simulink model "p1_standalone"  (R2014a)
settings: Solver=ode1  SolverMode=SingleTasking  StartTime=0  StopTime=36000  FixedStep=Ts  RelTol=1e-3
PreLoadFcn:
  | InitModel
  | make
InitFcn:
  | InitModel
  | make
values from neighbouring files (symbols this model uses):
  num = num+MTnum(m)    [Build_MtMuMy.m]
  Ts = 0.002    [DSC_Control_Analysis.m]    (also in DSC_Control_Analysis_Exp.m; DSC_Speed_Control_Analysis.m; EC_params_nissan.m; Ext_MPCPara.m = SSD.Ts)
undefined symbols (not defined in the file or in its folder): den, DiscIntNeverNeededParam, gpsins, gr, hal_filter_den, hal_filter_num, Igain_l, Igain_r, Imax_l, Imax_r, Ioff_l, Ioff_r, KB, Kd, KF, Ki, KJ, Kp, param, sglu
libraries: simulink x5, slrtlib x3, xpcdiamondlib x2, UserBlocks x1
(part 2 of 3)

== system p1_standalone/Hardware I//O/Input/GPS Velocity and Position ==
  Demux : Demux  Outputs=19
  GPS Velocity : S-Function  FunctionName=rs232_OEM4_MultiMode  Parameters=Ts, ModeSelect  EnableBusSupport=off
  Mux : Mux  Inputs=19
  Raw GPS : Outport
  wires:
  Mux/1 -> Raw GPS/1
  Demux/6 -> Mux/6  "Velocity Status Vel"
  Demux/7 -> Mux/7  "UTC DGPS"
  Demux/5 -> Mux/5  "Vert Speed"
  Demux/4 -> Mux/4  "Horiz Speed Direction"
  Demux/3 -> Mux/3  "Horiz Speed"
  Demux/2 -> Mux/2  "Latency Vel"
  Demux/1 -> Mux/1  "UTC Vel"
  Demux/19 -> Mux/19  "Latency"
  Demux/18 -> Mux/18  "Num Satellites"
  Demux/17 -> Mux/17  "Velocity z"
  Demux/16 -> Mux/16  "Velocity y"
  Demux/15 -> Mux/15  "Velocity x"
  Demux/14 -> Mux/14  "Velocity Solution Type"
  Demux/13 -> Mux/13  "Velocity Status"
  Demux/12 -> Mux/12  "Position z"
  Demux/11 -> Mux/11  "Postion y"
  Demux/10 -> Mux/10  "Position x"
  Demux/9 -> Mux/9  "Position Solution Type"
  Demux/8 -> Mux/8  "Position Status"
  GPS Velocity/1 -> Demux/1

== system p1_standalone/Hardware I//O/Input/Gearbox angle scaling ==
  raw gb angles : Inport
  Pot readings with wheels centered : Constant  Value=[ -1.73; -3.56 ]
  Sum : Sum  Inputs=|++  SaturateOnIntegerOverflow=on
  Volts/Rad : Gain  Gain=[1/ -1.31; 1/-1.34]  SaturateOnIntegerOverflow=on  OutDataTypeStr=Inherit: Same as input  ParamDataTypeStr=Inherit: Same as input
  gb angles : Outport
  wires:
  Volts/Rad/1 -> gb angles/1
  Pot readings with wheels centered/1 -> Sum/2
  raw gb angles/1 -> Sum/1
  Sum/1 -> Volts/Rad/1

== system p1_standalone/Hardware I//O/Input/Handwheel Scaling & Initialization ==
  Relative : Inport
  Absolute : Inport  Port=2
  Encoder Initialization : Subsystem
  Handwheel Gear Ratio : Gain  Gain=(60/18)*50  SaturateOnIntegerOverflow=on  OutDataTypeStr=Inherit: Same as input  ParamDataTypeStr=Inherit: Same as input
  Handwheel Sensor Fault Detection : Subsystem
  Harmonic Drive Gear Ratio : Gain  Gain=1/50  SaturateOnIntegerOverflow=on  OutDataTypeStr=Inherit: Same as input  ParamDataTypeStr=Inherit: Same as input
  Harmonic Drive Gear Ratio1 : Gain  Gain=1/50  SaturateOnIntegerOverflow=on  OutDataTypeStr=Inherit: Same as input  ParamDataTypeStr=Inherit: Same as input
  Sum : Sum  Inputs=|++
  encoder scaling : Gain  Gain=2*pi/(4*500)  SaturateOnIntegerOverflow=on  OutDataTypeStr=Inherit: Same as input  ParamDataTypeStr=Inherit: Same as input
  handwheel offset : Constant  Value=-1.29*pi/180*10
  Primary : Outport
  Secondary : Outport  Port=2
  Fault : Outport  Port=3
  wires:
  encoder scaling/1 -> Encoder Initialization/1(Relative Encoder)  "Primary"
  Handwheel Gear Ratio/1 -> Encoder Initialization/2(Absolute Encoder), Harmonic Drive Gear Ratio1/1
  Handwheel Sensor Fault Detection/3(Fault) -> Fault/1  "Encoder Fault Status"
  Encoder Initialization/1(Calibrated) -> Harmonic Drive Gear Ratio/1
  Handwheel Sensor Fault Detection/2(Secondary) -> Secondary/1  "Secondary"
  Harmonic Drive Gear Ratio/1 -> Handwheel Sensor Fault Detection/1(Relative)
  Relative/1 -> encoder scaling/1
  Absolute/1 -> Handwheel Gear Ratio/1
  Harmonic Drive Gear Ratio1/1 -> Handwheel Sensor Fault Detection/2(Absolute)
  handwheel offset/1 -> Sum/1
  Sum/1 -> Primary/1
  Handwheel Sensor Fault Detection/1(Primary) -> Sum/2  "Primary"

== system p1_standalone/Hardware I//O/Input/INS scaling ==
  raw INS : Inport
  Bus Creator : BusCreator  Inputs=6
  Demux : Demux  Outputs=9
  Gain : Gain  Gain=9.81  SaturateOnIntegerOverflow=on  OutDataTypeStr=Inherit: Same as input  ParamDataTypeStr=Inherit: Same as input
  Gain1 : Gain  Gain=1/.018  SaturateOnIntegerOverflow=on  OutDataTypeStr=Inherit: Same as input  ParamDataTypeStr=Inherit: Same as input
  Gain2 : Gain  Gain=1/.018  SaturateOnIntegerOverflow=on  OutDataTypeStr=Inherit: Same as input  ParamDataTypeStr=Inherit: Same as input
  Gain3 : Gain  Gain=9.81  SaturateOnIntegerOverflow=on  OutDataTypeStr=Inherit: Same as input  ParamDataTypeStr=Inherit: Same as input
  Gain4 : Gain  Gain=9.81  SaturateOnIntegerOverflow=on  OutDataTypeStr=Inherit: Same as input  ParamDataTypeStr=Inherit: Same as input
  Gain5 : Gain  Gain=1/.018  SaturateOnIntegerOverflow=on  OutDataTypeStr=Inherit: Same as input  ParamDataTypeStr=Inherit: Same as input
  Sum{,1..5} (6 alike) : Sum  Inputs=+-  SaturateOnIntegerOverflow=on  InputSameDT=on  OutDataTypeStr=Inherit: Same as first input
  deg to rad : Gain  Gain=pi/180  SaturateOnIntegerOverflow=on  OutDataTypeStr=Inherit: Same as input  ParamDataTypeStr=Inherit: Same as input
  INS : Outport
  wires:
  Demux/6 -> Sum2/2, Sum/2
  Demux/4 -> Sum2/1
  Demux/2 -> Sum3/1
  Demux/3 -> Sum3/2, Sum1/2
  Demux/1 -> Sum1/1
  Gain3/1 -> Bus Creator/2  "ax"
  Gain2/1 -> Bus Creator/3  "roll"
  Gain1/1 -> deg to rad/1  "yaw rate"
  Gain/1 -> Bus Creator/4  "ay"
  Sum3/1 -> Gain3/1
  Sum2/1 -> Gain2/1
  Sum1/1 -> Gain1/1
  Sum/1 -> Gain/1
  raw INS/1 -> Demux/1
  Gain5/1 -> Bus Creator/5  "pitch"
  Gain4/1 -> Bus Creator/6  "az"
  Sum5/1 -> Gain5/1
  Sum4/1 -> Gain4/1
  Demux/7 -> Sum5/1
  Demux/8 -> Sum4/1
  Demux/5 -> Sum/1
  Demux/9 -> Sum5/2, Sum4/2
  deg to rad/1 -> Bus Creator/1  "yaw"
  Bus Creator/1 -> INS/1

== system p1_standalone/Hardware I//O/Input/OEM4 wgsxyz2enu and status conversion ==
  raw GPS : Inport
  Bus Creator : BusCreator  Inputs=6
  Bus Creator1 : BusCreator  Inputs=6
  Bus Creator2 : BusCreator  Inputs=2
  Bus Creator3 : BusCreator  Inputs=6
  Bus Creator4 : BusCreator  Inputs=3
  Demux : Demux  Outputs=19
  Gain to make CW : Gain  Gain=-1
  Mode Select : Constant
  Switch : Switch  Threshold=0.5
  position preprocessing : Subsystem
  velocity preprocessing : Subsystem
  OEM4 Velocity : Outport
  OEM4 position : Outport  Port=2
  OEM4 other : Outport  Port=3
  OEM4 rawXYZ : Outport  Port=4
  wires:
  Switch/1 -> OEM4 Velocity/1
  Mode Select/1 -> Switch/2
  Bus Creator3/1 -> Switch/1
  Demux/6 -> Bus Creator3/6  "Velocity Solution Status"
  Demux/5 -> Bus Creator3/5  "Vertical Speed"
  Demux/4 -> Bus Creator3/4  "Horizontal Velocity Direction"
  Demux/3 -> Bus Creator3/3  "Horizontal Speed"
  Demux/2 -> Bus Creator3/2  "Latency"
  Demux/1 -> Bus Creator3/1  "UTC"
  Demux/19 -> Bus Creator1/2  "Latency"
  Gain to make CW/1 -> Bus Creator1/4  "Horizontal Velocity Direction"
  Demux/14 -> Bus Creator2/1  "Velocity Solution Type"
  Demux/18 -> Bus Creator2/2  "Number Of Satellites"
  Bus Creator2/1 -> OEM4 other/1
  Bus Creator/1 -> OEM4 position/1
  Demux/7 -> Bus Creator1/1, Bus Creator/1  "UTC"
  position preprocessing/3(Pos Up (z)) -> Bus Creator/6  "Pos Up (z)"
  position preprocessing/2(Pos N (y)) -> Bus Creator/5  "Pos N (y)"
  position preprocessing/1(Pos E (x)) -> Bus Creator/4  "Pos E (x)"
  Demux/8 -> Bus Creator/2  "Position Solution Status"
  Demux/9 -> Bus Creator/3  "Position Solution Type"
  Demux/10 -> position preprocessing/1(Pos x), Bus Creator4/1  "GPS_rawX"
  Demux/11 -> position preprocessing/2(Pos y), Bus Creator4/2  "GPS_rawY"
  Demux/12 -> position preprocessing/3(Pos z), Bus Creator4/3  "GPS_rawZ"
  velocity preprocessing/1(horizontal speed) -> Bus Creator1/3  "Horizontal Speed"
  velocity preprocessing/2(velocity direction) -> Gain to make CW/1  "Horizontal Velocity Direction"
  velocity preprocessing/3(vertical speed) -> Bus Creator1/5  "Vertical Speed"
  velocity preprocessing/4(velocity status) -> Bus Creator1/6  "Velocity Solution Status"
  Demux/13 -> velocity preprocessing/1(Vel status)
  Demux/15 -> velocity preprocessing/2(Vel x)  "Velocity Solution Type"
  Demux/16 -> velocity preprocessing/3(Vel y)
  Demux/17 -> velocity preprocessing/4(Vel z)
  Bus Creator1/1 -> Switch/3
  raw GPS/1 -> Demux/1
  Bus Creator4/1 -> OEM4 rawXYZ/1

== system p1_standalone/Hardware I//O/Input/Rear Wheel Speed Processing ==
  ticks : Inport
  Demux : Demux  Outputs=2
  Mux : Mux  Inputs=2
  Speed Calc : Subsystem  mask{range=65536}
      mask prompts: range "Wrap range"
      mask Display: disp(range);
  Speed Calc1 : Subsystem  mask{range=65536}
      mask prompts: range "Wrap range"
      mask Display: disp(range);
  de-quadrature : Gain  Gain=1/2
  ticks/sample : Outport
  wires:
  ticks/1 -> Demux/1
  Demux/1 -> Speed Calc/1(Distance)
  Speed Calc/1(Speed) -> Mux/1
  Demux/2 -> Speed Calc1/1(Distance)
  Speed Calc1/1(Speed) -> Mux/2
  Mux/1 -> de-quadrature/1
  de-quadrature/1 -> ticks/sample/1

== system p1_standalone/Hardware I//O/Input/Steering Motor Encoder Initialization ==
  Raw : Inport
  Potentiometer : Inport  Port=2
  Alignment : Inport  Port=3
  Demux : Demux  Outputs=2
  Demux1 : Demux  Outputs=2
  Left : Subsystem
  Mux : Mux  Inputs=2
  Right : Subsystem
  Sum1 : Sum  Inputs=++|
  Sum2 : Sum  Inputs=|++
  gearbox ratio : Gain  Gain=gr  SaturateOnIntegerOverflow=on  OutDataTypeStr=Inherit: Same as input  ParamDataTypeStr=Inherit: Same as input
  gearbox ratio1 : Gain  Gain=gr  SaturateOnIntegerOverflow=on  OutDataTypeStr=Inherit: Same as input  ParamDataTypeStr=Inherit: Same as input
  Angles : Outport
  Gearbox Angles : Outport  Port=2
  wires:
  Sum1/1 -> Gearbox Angles/1
  gearbox ratio1/1 -> Sum2/2
  Alignment/1 -> Sum1/1, gearbox ratio1/1
  Sum2/1 -> Angles/1
  Mux/1 -> Sum2/1
  Right/1(Calibrated) -> Mux/2
  gearbox ratio/1 -> Demux1/1
  Raw/1 -> Demux/1
  Potentiometer/1 -> Sum1/2, gearbox ratio/1
  Left/1(Calibrated) -> Mux/1
  Demux/1 -> Left/1(Encoder)
  Demux/2 -> Right/1(Encoder)
  Demux1/1 -> Left/2(Potentiometer)
  Demux1/2 -> Right/2(Potentiometer)

== system p1_standalone/Hardware I//O/Input/Subsystem1 ==
  In1 : Inport
  Constant : Constant
  Sum : Sum  Inputs=+-|
  Out1 : Outport
  wires:
  Sum/1 -> Out1/1
  In1/1 -> Sum/2
  Constant/1 -> Sum/1

== system p1_standalone/Hardware I//O/Input/Subsystem2 ==
  In1 : Inport
  Constant : Constant
  Sum : Sum  Inputs=+-|
  Out1 : Outport
  wires:
  Constant/1 -> Sum/1
  In1/1 -> Sum/2
  Sum/1 -> Out1/1

== system p1_standalone/Hardware I//O/Input/VSBC Analog Demux ==
  In : Inport
  Constant : Constant  Value=2.67
  Demux : Demux  Outputs=8
  Mux1 : Mux  Inputs=2
  Mux2 : Mux  Inputs=2
  Sum : Sum  Inputs=|+-
  T3 : Terminator
  Voltage to Rad : Gain  Gain=-(38.6)*(pi/180)
  PPS : Outport
  Motor Currents : Outport  Port=2
  HW Motor Current : Outport  Port=3
  HW Absolute Pot : Outport  Port=4
  Rear Load Cells : Outport  Port=5
  wires:
  Mux1/1 -> Motor Currents/1
  In/1 -> Demux/1
  Demux/7 -> Mux1/2
  Demux/6 -> Mux1/1
  Demux/3 -> HW Motor Current/1
  Demux/1 -> PPS/1
  Demux/8 -> T3/1
  Voltage to Rad/1 -> HW Absolute Pot/1
  Demux/4 -> Sum/1
  Sum/1 -> Voltage to Rad/1
  Constant/1 -> Sum/2
  Demux/2 -> Mux2/1
  Demux/5 -> Mux2/2
  Mux2/1 -> Rear Load Cells/1

== system p1_standalone/Hardware I//O/Input/current scaling ==
  volts : Inport
  Constant : Constant  Value=-5.39
  Sum : Sum  Inputs=|++  SaturateOnIntegerOverflow=on
  current scaling : Gain  Gain=30/7.5*3.3  SaturateOnIntegerOverflow=on  OutDataTypeStr=Inherit: Same as input  ParamDataTypeStr=Inherit: Same as input
  amps : Outport
  wires:
  volts/1 -> current scaling/1
  current scaling/1 -> Sum/1
  Sum/1 -> amps/1
  Constant/1 -> Sum/2

== system p1_standalone/Hardware I//O/Output/ConvertForce2Volt ==
  ForceDesired : Inport
  VoltDesired : Outport
  wires:
  ForceDesired/1 -> VoltDesired/1

== system p1_standalone/Sensor Data and Estimation/Nonlinear Observer/Normal Loads ==
  Vehicle States : Inport
  Bus Creator : BusCreator  Inputs=2
  Bus Selector1 : BusSelector  OutputSignals=Roll Angle,ayCG
  CG height : Constant  Value=0.49
  Fnf_nom : Constant  Value=param.m*9.81*param.b/(2*(param.a+param.b))
  Fnr_nom : Constant  Value=param.m*9.81*param.b/(2*(param.a+param.b))
  Front Mass : Constant  Value=param.m*param.b/(param.b+param.a)
  Left Normal Load : Sum  Inputs=+-
  Right Normal Load : Sum
  Roll Stiffness : Constant  Value=param.k_roll*0
  Saturation : Saturate  UpperLimit=deg2rad(8)  LowerLimit=-deg2rad(8)
  Track Width : Constant  Value=param.tw
  Track Width1 : Constant  Value=param.tw
  dFz : Sum
  dFz Ay Contribution : Product  Inputs=***/
  dFz Roll Contribution : Product  Inputs=**/
  Normal Loads : Outport
  wires:
  Bus Creator/1 -> Normal Loads/1
  Left Normal Load/1 -> Bus Creator/1  "Left"
  Right Normal Load/1 -> Bus Creator/2  "Right"
  Vehicle States/1 -> Bus Selector1/1
  Roll Stiffness/1 -> dFz Roll Contribution/1
  Bus Selector1/1 -> Saturation/1  "<Roll Angle>"
  Track Width1/1 -> dFz Roll Contribution/3
  Bus Selector1/2 -> dFz Ay Contribution/1  "<ayCG>"
  Front Mass/1 -> dFz Ay Contribution/2
  Fnf_nom/1 -> Left Normal Load/1
  dFz Roll Contribution/1 -> dFz/1
  dFz Ay Contribution/1 -> dFz/2
  dFz/1 -> Left Normal Load/2, Right Normal Load/1
  Fnr_nom/1 -> Right Normal Load/2
  Saturation/1 -> dFz Roll Contribution/2
  CG height/1 -> dFz Ay Contribution/3
  Track Width/1 -> dFz Ay Contribution/4

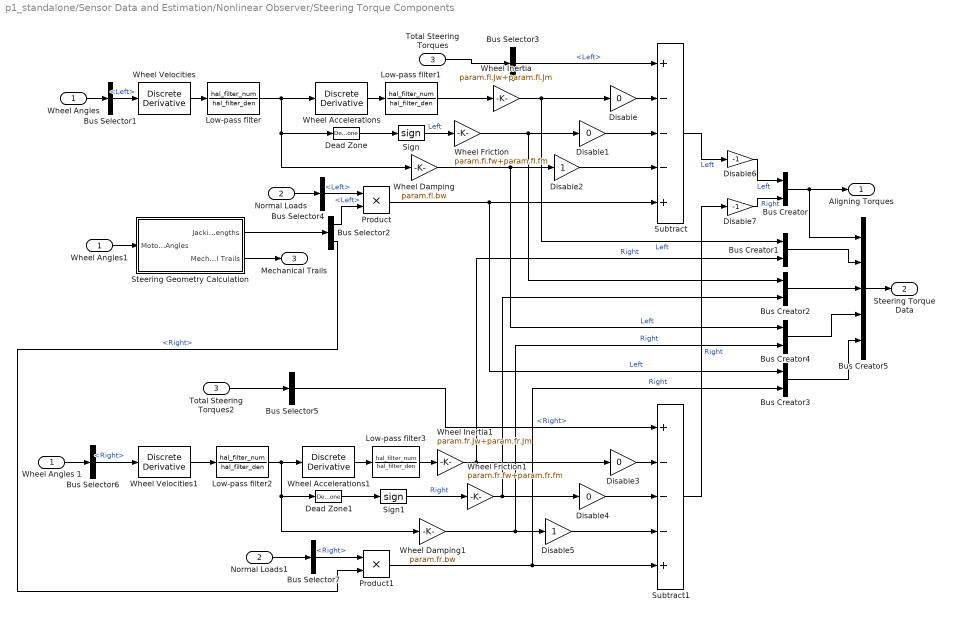
== system p1_standalone/Sensor Data and Estimation/Nonlinear Observer/Steering Torque Components ==
  Wheel Angles : Inport
  Normal Loads : Inport  Port=2
  Total Steering Torques : Inport  Port=3
  Bus Creator{,1..4} (5 alike) : BusCreator  Inputs=2
  Bus Creator5 : BusCreator  Inputs=5
  Bus Selector1 : BusSelector  OutputSignals=Left
  Bus Selector2 : BusSelector  OutputSignals=Left,Right
  Bus Selector3 : BusSelector  OutputSignals=Left
  Bus Selector4 : BusSelector  OutputSignals=Left
  Bus Selector5 : BusSelector  OutputSignals=Right
  Bus Selector6 : BusSelector  OutputSignals=Right
  Bus Selector7 : BusSelector  OutputSignals=Right
  Dead Zone : DeadZone  LowerValue=-0.03  UpperValue=0.03  SaturateOnIntegerOverflow=on
  Dead Zone1 : DeadZone  LowerValue=-0.03  UpperValue=0.03  SaturateOnIntegerOverflow=on
  Disable{,1,3..4} (4 alike) : Gain  Gain=0
  Disable2 : Gain
  Disable5 : Gain
  Disable6 : Gain  Gain=-1
  Disable7 : Gain  Gain=-1
  Low-pass filter{,1..3} (4 alike) : DiscreteTransferFcn  Numerator=hal_filter_num  Denominator=hal_filter_den  SampleTime=Ts
  Normal Loads1 : InportShadow  Port=2
  Product : Product  RndMeth=Zero
  Product1 : Product  RndMeth=Zero
  Sign : Signum
  Sign1 : Signum
  Steering Geometry Calculation : Subsystem
      mask init:
      | p1_params
      | nissan_steer_lookup_data
  Subtract : Sum  Inputs=+---+
  Subtract1 : Sum  Inputs=+---+
  Total Steering Torques2 : InportShadow  Port=3
  Wheel Accelerations : simulink/Discrete/Discrete Derivative  gainval=1.0  ICPrevScaledInput=0.0  InputProcessing=Inherited  OutMin=[]  OutMax=[]  OutDataType=sfix(16)  OutScaling=2^-10  DoSatur=off
  Wheel Accelerations1 : simulink/Discrete/Discrete Derivative  gainval=1.0  ICPrevScaledInput=0.0  InputProcessing=Inherited  OutMin=[]  OutMax=[]  OutDataType=sfix(16)  OutScaling=2^-10  DoSatur=off
  Wheel Angles 1 : InportShadow
  Wheel Angles1 : InportShadow
  Wheel Damping : Gain  Gain=param.fl.bw
  Wheel Damping1 : Gain  Gain=param.fr.bw
  Wheel Friction : Gain  Gain=param.fl.fw+param.fl.fm
  Wheel Friction1 : Gain  Gain=param.fr.fw+param.fr.fm
  Wheel Inertia : Gain  Gain=param.fl.Jw+param.fl.Jm
  Wheel Inertia1 : Gain  Gain=param.fr.Jw+param.fr.Jm
  Wheel Velocities : simulink/Discrete/Discrete Derivative  gainval=1.0  ICPrevScaledInput=0.0  InputProcessing=Inherited  OutMin=[]  OutMax=[]  OutDataType=sfix(16)  OutScaling=2^-10  DoSatur=off
  Wheel Velocities1 : simulink/Discrete/Discrete Derivative  gainval=1.0  ICPrevScaledInput=0.0  InputProcessing=Inherited  OutMin=[]  OutMax=[]  OutDataType=sfix(16)  OutScaling=2^-10  DoSatur=off
  Aligning Torques : Outport
  Steering Torque Data : Outport  Port=2
  Mechanical Trails : Outport  Port=3
  wires:
  Bus Selector3/1 -> Subtract/1  "<Left>"
  Wheel Velocities/1 -> Low-pass filter/1
  Steering Geometry Calculation/2(Mechanical Trails) -> Mechanical Trails/1
  Sign/1 -> Wheel Friction/1  "Left"
  Normal Loads/1 -> Bus Selector4/1
  Product/1 -> Bus Creator3/1, Subtract/5  "Left"
  Wheel Accelerations/1 -> Low-pass filter1/1
  Wheel Inertia/1 -> Bus Creator1/1, Disable/1  "Left"
  Wheel Angles/1 -> Bus Selector1/1
  Bus Selector5/1 -> Subtract1/1  "<Right>"
  Wheel Velocities1/1 -> Low-pass filter2/1
  Sign1/1 -> Wheel Friction1/1  "Right"
  Product1/1 -> Bus Creator3/2, Subtract1/5  "Right"
  Wheel Accelerations1/1 -> Low-pass filter3/1
  Wheel Inertia1/1 -> Bus Creator1/2, Disable3/1  "Right"
  Bus Selector1/1 -> Wheel Velocities/1  "<Left>"
  Bus Selector4/1 -> Product/1  "<Left>"
  Steering Geometry Calculation/1(Jacking Arm Lengths) -> Bus Selector2/1
  Bus Selector2/1 -> Product/2  "<Left>"
  Wheel Angles 1/1 -> Bus Selector6/1
  Bus Selector6/1 -> Wheel Velocities1/1  "<Right>"
  Bus Selector2/2 -> Product1/2  "<Right>"
  Normal Loads1/1 -> Bus Selector7/1
  Bus Selector7/1 -> Product1/1  "<Right>"
  Bus Creator/1 -> Aligning Torques/1, Bus Creator5/1
  Subtract/1 -> Disable6/1  "Left"
  Subtract1/1 -> Disable7/1  "Right"
  Wheel Damping/1 -> Bus Creator4/1, Disable2/1  "Left"
  Wheel Damping1/1 -> Bus Creator4/2, Disable5/1  "Right"
  Wheel Friction/1 -> Bus Creator2/1, Disable1/1
  Wheel Friction1/1 -> Bus Creator2/2, Disable4/1
  Bus Creator5/1 -> Steering Torque Data/1
  Bus Creator1/1 -> Bus Creator5/2
  Bus Creator2/1 -> Bus Creator5/3
  Bus Creator4/1 -> Bus Creator5/4
  Bus Creator3/1 -> Bus Creator5/5
  Disable/1 -> Subtract/2
  Disable1/1 -> Subtract/3
  Disable2/1 -> Subtract/4
  Disable3/1 -> Subtract1/2
  Disable4/1 -> Subtract1/3
  Disable5/1 -> Subtract1/4
  Total Steering Torques2/1 -> Bus Selector5/1
  Total Steering Torques/1 -> Bus Selector3/1
  Disable6/1 -> Bus Creator/1  "Left"
  Disable7/1 -> Bus Creator/2  "Right"
  Low-pass filter/1 -> Wheel Damping/1, Dead Zone/1, Wheel Accelerations/1
  Low-pass filter1/1 -> Wheel Inertia/1
  Low-pass filter2/1 -> Wheel Accelerations1/1, Wheel Damping1/1, Dead Zone1/1
  Low-pass filter3/1 -> Wheel Inertia1/1
  Dead Zone/1 -> Sign/1
  Dead Zone1/1 -> Sign1/1
  Wheel Angles1/1 -> Steering Geometry Calculation/1(Motor Angles)

== system p1_standalone/Sensor Data and Estimation/Steering Kinematics/Steer Torque Calculation ==
  Motor Angles : Inport
  Load Cells : Inport  Port=2
  Bus Creator : BusCreator  Inputs=2
  Demux : Demux  Outputs=2
  Demux1 : Demux  Outputs=2
  Left Arm Length Look-up : Lookup_n-D  NumberOfTableDimensions=1  BreakpointsForDimension1=sglu.fl.ma  Table=sglu.fl.lc  InternalRulePriority=Speed  SaturateOnIntegerOverflow=on  InputSameDT=on
  Left Steering Ratio : Gain  Gain=1/param.fl.gr  SaturateOnIntegerOverflow=on  OutDataTypeStr=Inherit: Same as input  ParamDataTypeStr=Inherit: Same as input
  Product : Product  RndMeth=Zero
  Product1 : Product  RndMeth=Zero
  Right Arm Length Look-up : Lookup_n-D  NumberOfTableDimensions=1  BreakpointsForDimension1=sglu.fr.ma  Table=sglu.fr.lc  InternalRulePriority=Speed  SaturateOnIntegerOverflow=on  InputSameDT=on
  Right Steering Ratio : Gain  Gain=1/param.fr.gr  SaturateOnIntegerOverflow=on  OutDataTypeStr=Inherit: Same as input  ParamDataTypeStr=Inherit: Same as input
  Steer Torques : Outport
  wires:
  Motor Angles/1 -> Demux/1
  Bus Creator/1 -> Steer Torques/1
  Demux/1 -> Left Steering Ratio/1
  Demux/2 -> Right Steering Ratio/1
  Left Steering Ratio/1 -> Left Arm Length Look-up/1
  Right Steering Ratio/1 -> Right Arm Length Look-up/1
  Load Cells/1 -> Demux1/1
  Demux1/2 -> Product1/2
  Demux1/1 -> Product/2
  Left Arm Length Look-up/1 -> Product/1
  Right Arm Length Look-up/1 -> Product1/1
  Product1/1 -> Bus Creator/2  "Right"
  Product/1 -> Bus Creator/1  "Left"

== system p1_standalone/Sensor Data and Estimation/Steering Kinematics/Steering Angle Calculation ==
  Motor Angles : Inport
  Bus Creator : BusCreator  Inputs=2
  Demux : Demux  Outputs=2
  Left Steer Angle Look-up : Lookup_n-D  NumberOfTableDimensions=1  BreakpointsForDimension1=sglu.fl.ma  Table=sglu.fl.sa  InternalRulePriority=Speed  SaturateOnIntegerOverflow=on  InputSameDT=on
  Left Steering Ratio : Gain  Gain=1/param.fl.gr  SaturateOnIntegerOverflow=on  OutDataTypeStr=Inherit: Same as input  ParamDataTypeStr=Inherit: Same as input
  Right Steer Angle Look-up : Lookup_n-D  NumberOfTableDimensions=1  BreakpointsForDimension1=sglu.fr.ma  Table=sglu.fr.sa  InternalRulePriority=Speed  SaturateOnIntegerOverflow=on  InputSameDT=on
  Right Steering Ratio : Gain  Gain=1/param.fr.gr  SaturateOnIntegerOverflow=on  OutDataTypeStr=Inherit: Same as input  ParamDataTypeStr=Inherit: Same as input
  Steer Angles : Outport
  wires:
  Motor Angles/1 -> Demux/1
  Bus Creator/1 -> Steer Angles/1
  Demux/1 -> Left Steering Ratio/1
  Demux/2 -> Right Steering Ratio/1
  Left Steering Ratio/1 -> Left Steer Angle Look-up/1
  Right Steering Ratio/1 -> Right Steer Angle Look-up/1
  Left Steer Angle Look-up/1 -> Bus Creator/1  "Left"
  Right Steer Angle Look-up/1 -> Bus Creator/2  "Right"

== system p1_standalone/Sensor Data and Estimation/Vehicle State Estimator/Select: Yaw Rate ==
  In1 : Inport
  Gain : Gain  Gain=K  Multiplication=Matrix(K*u)  SaturateOnIntegerOverflow=on  OutDataTypeStr=Inherit: Same as input  ParamDataTypeStr=Inherit: Same as input
  Out1 : Outport
  wires:
  Gain/1 -> Out1/1
  In1/1 -> Gain/1

== system p1_standalone/Sensor Data and Estimation/Vehicle State Estimator/state estimation ==
  gps : Inport
  ins : Inport  Port=2
  Bus Creator : BusCreator  Inputs=21
  DegtoRad{1..7} (7 alike) : Gain  Gain=pi/180
  Roll Gyro Sf : Constant
  Super Filter : Subsystem
  Filter Output : Outport
  wires:
  Super Filter/8(Vx) -> Bus Creator/9  "Vx"
  Super Filter/9(ax bias) -> Bus Creator/10  "ax bias"
  Super Filter/12(VyCG) -> Bus Creator/12  "VyCG"
  Super Filter/13(axCG) -> Bus Creator/11  "axCG"
  Bus Creator/1 -> Filter Output/1
  DegtoRad2/1 -> Bus Creator/1  "Yaw Angle"
  Super Filter/1(Yaw Angle) -> DegtoRad2/1  "Yaw Angle"
  Super Filter/4(Corr Yaw Rate) -> DegtoRad1/1  "Yaw Rate"
  DegtoRad1/1 -> Bus Creator/4  "Yaw Rate"
  Super Filter/5(Roll Angle) -> DegtoRad3/1  "Roll Angle"
  DegtoRad3/1 -> Bus Creator/5  "Roll Angle"
  Super Filter/7(Corr Roll Rate) -> DegtoRad4/1  "Roll Rate"
  DegtoRad4/1 -> Bus Creator/8  "Roll Rate"
  DegtoRad5/1 -> Bus Creator/3  "Yaw Gyro Bias"
  Super Filter/3(Yaw Gyro Bias) -> DegtoRad5/1  "Yaw Gyro Bias"
  Super Filter/6(Roll Gyro Bias) -> DegtoRad6/1  "Roll Gyro Bias"
  DegtoRad6/1 -> Bus Creator/7  "Roll Gyro Bias"
  DegtoRad7/1 -> Bus Creator/15  "Sideslip"
  Super Filter/2(Yaw Gyro Sf) -> Bus Creator/2  "Yaw Gyro Sf"
  Super Filter/16(Pos E) -> Bus Creator/16  "Pos E"
  Super Filter/17(OEM4 Delay) -> Bus Creator/18  "OEM4 Delay"
  Super Filter/18(Beeline Delay) -> Bus Creator/19  "Beeline Delay"
  Super Filter/19(OEM4 Update Pulse) -> Bus Creator/20  "OEM4 Update"
  Super Filter/20(Beeline Update Pulse) -> Bus Creator/21  "Beeline Update"
  Roll Gyro Sf/1 -> Bus Creator/6  "Roll Gyro Sf"
  gps/1 -> Super Filter/1(GPS)
  ins/1 -> Super Filter/2(INS)
  Super Filter/11(Sideslip) -> DegtoRad7/1  "Sideslip"
  Super Filter/10(ay bias) -> Bus Creator/13  "ay bias"
  Super Filter/14(ayCG) -> Bus Creator/14  "ayCG"
  Super Filter/15(Pos N) -> Bus Creator/17  "Pos N"

== system p1_standalone/Hardware I//O/Input/Handwheel Scaling & Initialization/Encoder Initialization ==
  Relative Encoder : Inport
  Absolute Encoder : Inport  Port=2
  Encoder Initializer : S-Function  FunctionName=encoderinit  Parameters=sampleTime,firstDelay,secondDelay  EnableBusSupport=off  mask{sampleTime=Ts, firstDelay=.1, secondDelay=.2}
      mask prompts: sampleTime "Sample time"; firstDelay "First calibration time"; secondDelay "Second calibration time"
      mask Display:
      | port_label('input',1,'Unwrapped');
      | port_label('input',2,'Raw');
      | port_label('input',3,'Absolute');
      | port_label('output',1,'Calibrated');
  Unwrapper : S-Function  FunctionName=unwrapper  Parameters=Ts,2*pi  EnableBusSupport=off
      mask Display: disp('2*pi')
  Calibrated : Outport
  wires:
  Absolute Encoder/1 -> Encoder Initializer/3
  Unwrapper/1 -> Encoder Initializer/1
  Relative Encoder/1 -> Unwrapper/1, Encoder Initializer/2
  Encoder Initializer/1 -> Calibrated/1

== system p1_standalone/Hardware I//O/Input/Handwheel Scaling & Initialization/Handwheel Sensor Fault Detection ==
  Relative : Inport
  Absolute : Inport  Port=2
  Descision Logic : Subsystem
  Enable Timer : Subsystem
  Fault Detection1 : Subsystem
  Ground : Ground
  Switch Over : Subsystem
  Terminator : Terminator
  Primary : Outport
  Secondary : Outport  Port=2
  Fault : Outport  Port=3
  wires:
  Relative/1 -> Switch Over/1(Relative), Fault Detection1/1(Relative)
  Fault Detection1/2(Jump) -> Descision Logic/2(Jump)
  Absolute/1 -> Switch Over/3(Absolute), Fault Detection1/2(Absolute)
  Fault Detection1/1(Disparity) -> Descision Logic/1(Disparity)
  Descision Logic/1(Best Bet) -> Terminator/1
  Switch Over/1(Primary) -> Primary/1
  Descision Logic/2(Fault) -> Fault/1
  Switch Over/2(Secondary) -> Secondary/1
  Enable Timer/1(Enable) -> Descision Logic/5(Enable)
  Fault Detection1/4(Partially Frozen) -> Descision Logic/4(Partially Frozen)
  Fault Detection1/3(Frozen) -> Descision Logic/3(Frozen)
  Ground/1 -> Switch Over/2(Chooser)

== system p1_standalone/Hardware I//O/Input/OEM4 wgsxyz2enu and status conversion/position preprocessing ==
  Pos x : Inport
  Pos y : Inport  Port=2
  Pos z : Inport  Port=3
  Mux1 : Mux  Inputs=3
  Position Converter : Subsystem
  Reference : Constant  Value="[ -2.693164268260626  -4.297082318497891   3.855183392965450]*1e6"
  Reference1 : Constant  Value=0
  Reference2 : Constant  Value=0
  Reference3 : Constant  Value=0
  Sum : Sum  Inputs=|++  SaturateOnIntegerOverflow=on
  Sum1 : Sum  Inputs=|++  SaturateOnIntegerOverflow=on
  Sum2 : Sum  Inputs=|++  SaturateOnIntegerOverflow=on
  Pos E (x) : Outport
  Pos N (y) : Outport  Port=2
  Pos Up (z) : Outport  Port=3
  wires:
  Sum2/1 -> Pos Up (z)/1
  Reference3/1 -> Sum2/2
  Sum1/1 -> Pos E (x)/1
  Reference2/1 -> Sum1/1
  Position Converter/1(East(x)) -> Sum1/2
  Sum/1 -> Pos N (y)/1
  Reference1/1 -> Sum/2
  Position Converter/2(North(Y)) -> Sum/1
  Pos x/1 -> Mux1/1
  Pos y/1 -> Mux1/2
  Pos z/1 -> Mux1/3
  Mux1/1 -> Position Converter/1(xyz)
  Reference/1 -> Position Converter/2(reference)
  Position Converter/3(Up) -> Sum2/1

== system p1_standalone/Hardware I//O/Input/OEM4 wgsxyz2enu and status conversion/velocity preprocessing ==
  note: vel N
  note: vel E
  Vel status : Inport
  Vel x : Inport  Port=2
  Vel y : Inport  Port=3
  Vel z : Inport  Port=4
  CCW from N : Constant  Value=90
  Comparison to .1 : RelationalOperator  Operator===  InputSameDT=on
  Mux : Mux  Inputs=2
  Mux1 : Mux  Inputs=3
  Reference : Constant  Value="[ -2.700929934500000E6  -4.291896551500000E6  3.855544188700000E6]"
  Sum : Sum  Inputs=|+-  SaturateOnIntegerOverflow=on
  Velocity Converter : Subsystem
  gain : Gain  Gain=3  SaturateOnIntegerOverflow=on  OutDataTypeStr=Inherit: Same as input  ParamDataTypeStr=Inherit: Same as input
  good : Constant  Value=0.1
  rad to deg : Gain  Gain=180/pi  SaturateOnIntegerOverflow=on  OutDataTypeStr=Inherit: Same as input  ParamDataTypeStr=Inherit: Same as input
  velocity direction (CCW from E) : Fcn  Expr=atan2(u[2],u[1])
  velocity magnitude : Fcn  Expr=sqrt(u[1]^2+u[2]^2)
  horizontal speed : Outport
  velocity direction : Outport  Port=2
  vertical speed : Outport  Port=3
  velocity status : Outport  Port=4
  wires:
  Vel x/1 -> Mux1/1
  Vel y/1 -> Mux1/2
  Vel z/1 -> Mux1/3
  Velocity Converter/2(North(Y)) -> Mux/2
  Vel status/1 -> Comparison to .1/1
  Velocity Converter/3(Up) -> vertical speed/1
  Velocity Converter/1(East(x)) -> Mux/1
  Mux1/1 -> Velocity Converter/1(xyz)
  Reference/1 -> Velocity Converter/2(reference)
  gain/1 -> velocity status/1
  Comparison to .1/1 -> gain/1
  good/1 -> Comparison to .1/2
  Sum/1 -> velocity direction/1
  velocity magnitude/1 -> horizontal speed/1
  CCW from N/1 -> Sum/2
  rad to deg/1 -> Sum/1
  velocity direction (CCW from E)/1 -> rad to deg/1
  Mux/1 -> velocity magnitude/1, velocity direction (CCW from E)/1

== system p1_standalone/Hardware I//O/Input/Rear Wheel Speed Processing/Speed Calc ==
  Distance : Inport
  Clock : Clock
  Difference : DiscreteTransferFcn  Numerator=[1 -1]  Denominator=[1 0]
  Mux : Mux  Inputs=2
  Unwrapping : Fcn  Expr=((u<=-range/2) - (u>=range/2)) * range + u
  Zero @ t=0; normal otherwise : Fcn  Expr=(u(2)>0) * u(1)
  Speed : Outport
  wires:
  Zero @ t=0; normal otherwise/1 -> Speed/1
  Mux/1 -> Zero @ t=0; normal otherwise/1
  Clock/1 -> Mux/2
  Difference/1 -> Unwrapping/1
  Distance/1 -> Difference/1
  Unwrapping/1 -> Mux/1

== system p1_standalone/Hardware I//O/Input/Rear Wheel Speed Processing/Speed Calc1 ==
  Distance : Inport
  Clock : Clock
  Difference : DiscreteTransferFcn  Numerator=[1 -1]  Denominator=[1 0]
  Mux : Mux  Inputs=2
  Unwrapping : Fcn  Expr=((u<=-range/2) - (u>=range/2)) * range + u
  Zero @ t=0; normal otherwise : Fcn  Expr=(u(2)>0) * u(1)
  Speed : Outport
  wires:
  Unwrapping/1 -> Mux/1
  Distance/1 -> Difference/1
  Difference/1 -> Unwrapping/1
  Clock/1 -> Mux/2
  Mux/1 -> Zero @ t=0; normal otherwise/1
  Zero @ t=0; normal otherwise/1 -> Speed/1

== system p1_standalone/Hardware I//O/Input/Steering Motor Encoder Initialization/Left ==
  Encoder : Inport
  Potentiometer : Inport  Port=2
  Encoder Initializer : S-Function  FunctionName=encoderinit  Parameters=sampleTime,firstDelay,secondDelay  EnableBusSupport=off  mask{sampleTime=Ts, firstDelay=.1, secondDelay=.2}
      mask prompts: sampleTime "Sample time"; firstDelay "First calibration time"; secondDelay "Second calibration time"
      mask Display:
      | port_label('input',1,'Unwrapped');
      | port_label('input',2,'Raw');
      | port_label('input',3,'Pot');
      | port_label('output',1,'Calibrated');
  Unwrapper : S-Function  FunctionName=unwrapper  Parameters=Ts,2*pi  EnableBusSupport=off
      mask Display: disp('2*pi')
  Calibrated : Outport
  wires:
  Encoder Initializer/1 -> Calibrated/1
  Encoder/1 -> Encoder Initializer/2, Unwrapper/1
  Unwrapper/1 -> Encoder Initializer/1
  Potentiometer/1 -> Encoder Initializer/3

== system p1_standalone/Hardware I//O/Input/Steering Motor Encoder Initialization/Right ==
  Encoder : Inport
  Potentiometer : Inport  Port=2
  Encoder Initializer : S-Function  FunctionName=encoderinit  Parameters=sampleTime,firstDelay,secondDelay  EnableBusSupport=off  mask{sampleTime=Ts, firstDelay=.1, secondDelay=.2}
      mask prompts: sampleTime "Sample time"; firstDelay "First calibration time"; secondDelay "Second calibration time"
      mask Display:
      | port_label('input',1,'Unwrapped');
      | port_label('input',2,'Raw');
      | port_label('input',3,'Pot');
      | port_label('output',1,'Calibrated');
  Unwrapper : S-Function  FunctionName=unwrapper  Parameters=Ts,2*pi  EnableBusSupport=off
      mask Display: disp('2*pi')
  Calibrated : Outport
  wires:
  Potentiometer/1 -> Encoder Initializer/3
  Encoder Initializer/1 -> Calibrated/1
  Unwrapper/1 -> Encoder Initializer/1
  Encoder/1 -> Encoder Initializer/2, Unwrapper/1

== system p1_standalone/Sensor Data and Estimation/Nonlinear Observer/Steering Torque Components/Steering Geometry Calculation ==
  Motor Angles : Inport
  Bus Creator : BusCreator  Inputs=2
  Bus Creator1 : BusCreator  Inputs=2
  Bus Selector1 : BusSelector  OutputSignals=Left,Right
  Left Steer Angle Look-up : Lookup_n-D  NumberOfTableDimensions=1  BreakpointsForDimension1=sglu.fl.sa  Table=sglu.fl.ja  InternalRulePriority=Speed  SaturateOnIntegerOverflow=on  InputSameDT=on
  Left Steer Angle Look-up1 : Lookup_n-D  NumberOfTableDimensions=1  BreakpointsForDimension1=sglu.fl.sa  Table=sglu.fl.mt  InternalRulePriority=Speed  SaturateOnIntegerOverflow=on  InputSameDT=on
  Right Steer Angle Look-up : Lookup_n-D  NumberOfTableDimensions=1  BreakpointsForDimension1=sglu.fr.sa  Table=sglu.fr.ja  InternalRulePriority=Speed  SaturateOnIntegerOverflow=on  InputSameDT=on
  Right Steer Angle Look-up1 : Lookup_n-D  NumberOfTableDimensions=1  BreakpointsForDimension1=sglu.fr.sa  Table=sglu.fr.mt  InternalRulePriority=Speed  SaturateOnIntegerOverflow=on  InputSameDT=on
  Jacking Arm Lengths : Outport
  Mechanical Trails : Outport  Port=2
  wires:
  Motor Angles/1 -> Bus Selector1/1
  Bus Creator/1 -> Jacking Arm Lengths/1
  Left Steer Angle Look-up/1 -> Bus Creator/1  "Left"
  Right Steer Angle Look-up/1 -> Bus Creator/2  "Right"
  Bus Creator1/1 -> Mechanical Trails/1
  Left Steer Angle Look-up1/1 -> Bus Creator1/1  "Left"
  Bus Selector1/1 -> Left Steer Angle Look-up/1, Left Steer Angle Look-up1/1  "<Left>"
  Bus Selector1/2 -> Right Steer Angle Look-up/1, Right Steer Angle Look-up1/1  "<Right>"
  Right Steer Angle Look-up1/1 -> Bus Creator1/2  "Right"

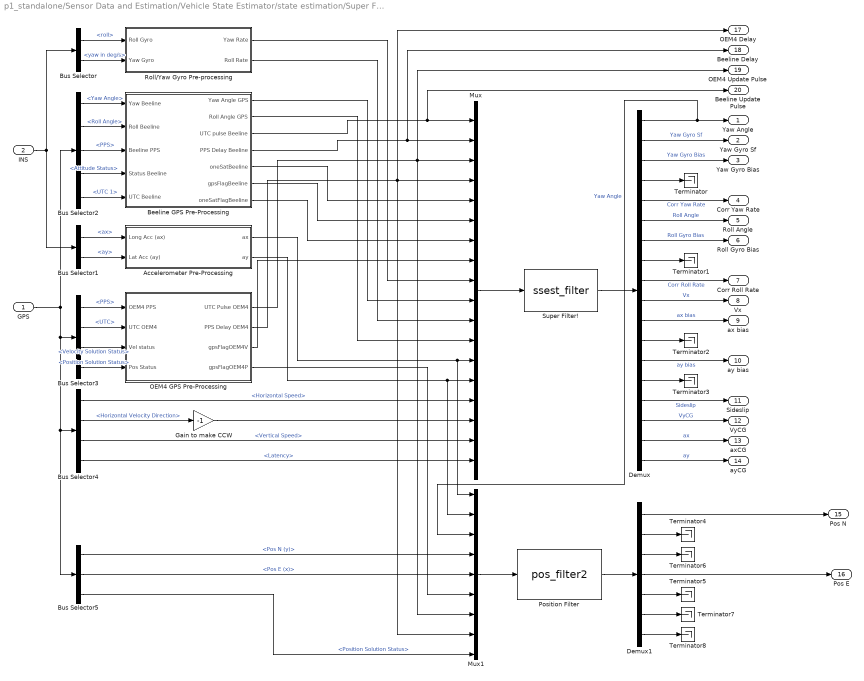
== system p1_standalone/Sensor Data and Estimation/Vehicle State Estimator/state estimation/Super Filter ==
  GPS : Inport
  INS : Inport  Port=2
  Accelerometer Pre-Processing : Subsystem
  Beeline GPS Pre-Processing : Subsystem
      mask init:
      | % this code sets the max delay to the value
      | % in ssest_params or to 1000000x that value
      | % if we're in pre-recorded data mode
      | 
      | flag=sum(strcmp(find_system(gcs),[gcs '/Pre-recorded Data']));
      | 
      | if flag==1; % this is pre-recorded mode, set 1000000x larger delay
      |     set_param([gcb '/Delay function'],'Parameters','gpsins.maxbeelinedelayoffline, Ts')
      | else;
      |     set_param([gcb '/Delay function'],'Parameters','gpsins.maxbeelinedelay, Ts')
      | end;
  Bus Selector : BusSelector  OutputSignals=roll,yaw in deg/s
  Bus Selector1 : BusSelector  OutputSignals=ax,ay
  Bus Selector2 : BusSelector  OutputSignals=Beeline.Yaw Angle,Beeline.Roll Angle,PPS,Beeline.Attitude Status,Beeline.UTC 1
  Bus Selector3 : BusSelector  OutputSignals=PPS,OEM4 Velocity.UTC,OEM4 Velocity.Velocity Solution Status,OEM4 Position.Position Solution Status
  Bus Selector4 : BusSelector  OutputSignals=OEM4 Velocity.Horizontal Speed,OEM4 Velocity.Horizontal Velocity Direction,OEM4 Velocity.Vertical Speed,OEM4 Velocity.Latency
  Bus Selector5 : BusSelector  OutputSignals=OEM4 Position.Pos N (y),OEM4 Position.Pos E (x),OEM4 Position.Position Solution Status
  Demux : Demux  Outputs=[1 1 1 9 1 1 1 4 1 1 1 1 1 16 1 1 1 1]
  Demux1 : Demux  Outputs=[1 1 1 1 1 1 36]
  Gain to make CCW : Gain  Gain=-1
  Mux : Mux  Inputs=18
  Mux1 : Mux  Inputs=9
  OEM4 GPS Pre-Processing : Subsystem
      mask init:
      | % this code sets the max delay to the value
      | % in ssest_params or to 1000000x that value
      | % if we're in pre-recorded data mode
      | 
      | flag=sum(strcmp(find_system(gcs),[gcs '/Pre-recorded Data']));
      | 
      | if flag==1; % this is pre-recorded mode, set 1000000x larger delay
      |     set_param([gcb '/Delay function'],'Parameters','gpsins.maxoem4delayoffline, Ts')
      | else;
      |     set_param([gcb '/Delay function'],'Parameters','gpsins.maxoem4delay, Ts')
      | end;
  Position Filter : S-Function  FunctionName=pos_filter2  Parameters=gpsins.initPosE, gpsins.initPosN  EnableBusSupport=off
  Roll/Yaw Gyro Pre-processing : Subsystem
  Super Filter! : S-Function  FunctionName=ssest_filter  Parameters=gpsins.init_state_hdg, gpsins.init_cov_hdg, gpsins.init_state_roll, gpsins.init_cov_roll, gpsins.init_state_vel, gpsins.init_cov_vel, gpsins.hdgfilter.sens_var, gpsins.hdgfilter.timeconst1, gpsins.hdgfilter.timeconst2, gpsins.hdgfilter.msr_var, gpsins.hdgfilter.init_sf_var, gpsins.diff_yaw, gpsins.rollfilter.sens_var, gpsins.rollfilter.timeconst, gpsins.rollfilter.msr_var, gpsins.diff_roll, gpsins.splitbeelinedelay, gpsins.dist_sensor, gpsins.height_sensor, gpsins.h_gps_ant, gpsins.l_gps_ant, gpsins.velfilter.sens1_var, gpsins.velfilter.sens2_var, gpsins.velfilter.timeconst1, gpsins.velfilter.timeconst2, gpsins.velfilter.msr1_var, gpsins.velfilter.msr2_var, gpsins.diff_vel_x, gpsins.diff_vel_y, gpsins.num_grade_avg, Ts  EnableBusSupport=off
  Terminator{,1..8} (9 alike) : Terminator
  Yaw Angle : Outport
  Yaw Gyro Sf : Outport  Port=2
  Yaw Gyro Bias : Outport  Port=3
  Corr Yaw Rate : Outport  Port=4
  Roll Angle : Outport  Port=5
  Roll Gyro Bias : Outport  Port=6
  Corr Roll Rate : Outport  Port=7
  Vx : Outport  Port=8
  ax bias : Outport  Port=9
  ay bias : Outport  Port=10
  Sideslip : Outport  Port=11
  VyCG : Outport  Port=12
  axCG : Outport  Port=13
  ayCG : Outport  Port=14
  Pos N : Outport  Port=15
  Pos E : Outport  Port=16
  OEM4 Delay : Outport  Port=17
  Beeline Delay : Outport  Port=18
  OEM4 Update Pulse : Outport  Port=19
  Beeline Update Pulse : Outport  Port=20
  wires:
  Beeline GPS Pre-Processing/3(UTC pulse Beeline) -> Mux/1, Beeline Update Pulse/1
  Beeline GPS Pre-Processing/4(PPS Delay Beeline) -> Mux/2, Beeline Delay/1
  Beeline GPS Pre-Processing/5(oneSatBeeline) -> Mux/5
  Beeline GPS Pre-Processing/6(gpsFlagBeeline) -> Mux/6
  Beeline GPS Pre-Processing/7(oneSatFlagBeeline) -> Mux/7
  Roll/Yaw Gyro Pre-processing/1(Yaw Rate) -> Mux/9
  Beeline GPS Pre-Processing/1(Yaw Angle GPS) -> Mux/10
  Roll/Yaw Gyro Pre-processing/2(Roll Rate) -> Mux/11
  Beeline GPS Pre-Processing/2(Roll Angle GPS) -> Mux/12
  Accelerometer Pre-Processing/1(ax) -> Mux/13, Mux1/1
  Accelerometer Pre-Processing/2(ay) -> Mux/14, Mux1/2
  Mux/1 -> Super Filter!/1
  Super Filter!/1 -> Demux/1
  Demux/1 -> Yaw Angle/1, Mux1/3  "Yaw Angle"
  Demux/2 -> Yaw Gyro Sf/1  "Yaw Gyro Sf"
  Demux/3 -> Yaw Gyro Bias/1  "Yaw Gyro Bias"
  Demux/4 -> Terminator/1
  Demux/5 -> Corr Yaw Rate/1  "Corr Yaw Rate"
  Demux/6 -> Roll Angle/1  "Roll Angle"
  Demux/7 -> Roll Gyro Bias/1  "Roll Gyro Bias"
  Demux/8 -> Terminator1/1
  Demux/9 -> Corr Roll Rate/1  "Corr Roll Rate"
  Demux/10 -> Vx/1  "Vx"
  Demux/11 -> ax bias/1  "ax bias"
  Demux/12 -> Terminator2/1
  Demux/13 -> ay bias/1  "ay bias"
  Demux/14 -> Terminator3/1
  Demux/15 -> Sideslip/1  "Sideslip"
  Demux/16 -> VyCG/1  "VyCG"
  Demux/17 -> axCG/1  "ax"
  Demux/18 -> ayCG/1  "ay"
  Mux1/1 -> Position Filter/1
  Position Filter/1 -> Demux1/1
  Demux1/2 -> Terminator4/1
  Demux1/3 -> Terminator6/1
  Demux1/5 -> Terminator5/1
  Demux1/6 -> Terminator7/1
  Demux1/7 -> Terminator8/1
  OEM4 GPS Pre-Processing/1(UTC Pulse OEM4) -> Mux/3, OEM4 Update Pulse/1, Mux1/7
  OEM4 GPS Pre-Processing/2(PPS Delay OEM4) -> Mux/4, OEM4 Delay/1, Mux1/8
  OEM4 GPS Pre-Processing/3(gpsFlagOEM4V) -> Mux/8
  INS/1 -> Bus Selector/1, Bus Selector1/1
  Bus Selector/1 -> Roll/Yaw Gyro Pre-processing/1(Roll Gyro)  "<roll>"
  Bus Selector/2 -> Roll/Yaw Gyro Pre-processing/2(Yaw Gyro)  "<yaw in deg/s>"
  Bus Selector1/1 -> Accelerometer Pre-Processing/1(Long Acc (ax))  "<ax>"
  Bus Selector1/2 -> Accelerometer Pre-Processing/2(Lat Acc (ay))  "<ay>"
  GPS/1 -> Bus Selector2/1, Bus Selector3/1, Bus Selector4/1, Bus Selector5/1
  Bus Selector2/1 -> Beeline GPS Pre-Processing/1(Yaw Beeline)  "<Yaw Angle>"
  Bus Selector2/2 -> Beeline GPS Pre-Processing/2(Roll Beeline)  "<Roll Angle>"
  Bus Selector2/3 -> Beeline GPS Pre-Processing/3("Beeline PPS ")  "<PPS>"
  Bus Selector2/4 -> Beeline GPS Pre-Processing/4(Status Beeline)  "<Attitude Status>"
  Bus Selector2/5 -> Beeline GPS Pre-Processing/5(UTC Beeline)  "<UTC 1>"
  Bus Selector3/1 -> OEM4 GPS Pre-Processing/1(OEM4 PPS)  "<PPS>"
  Bus Selector3/2 -> OEM4 GPS Pre-Processing/2(UTC OEM4)  "<UTC>"
  Bus Selector3/3 -> OEM4 GPS Pre-Processing/3(Vel status)  "<Velocity Solution Status>"
  Bus Selector3/4 -> OEM4 GPS Pre-Processing/4(Pos Status)  "<Position Solution Status>"
  Bus Selector4/1 -> Mux/15  "<Horizontal Speed>"
  Bus Selector4/2 -> Gain to make CCW/1  "<Horizontal Velocity Direction>"
  Bus Selector4/3 -> Mux/17  "<Vertical Speed>"
  Bus Selector4/4 -> Mux/18  "<Latency>"
  Bus Selector5/1 -> Mux1/4  "<Pos N (y)>"
  Bus Selector5/2 -> Mux1/5  "<Pos E (x)>"
  OEM4 GPS Pre-Processing/4(gpsFlagOEM4P) -> Mux1/6
  Gain to make CCW/1 -> Mux/16
  Demux1/1 -> Pos N/1
  Demux1/4 -> Pos E/1
  Bus Selector5/3 -> Mux1/9  "<Position Solution Status>"

== system p1_standalone/Hardware I//O/Input/Handwheel Scaling & Initialization/Handwheel Sensor Fault Detection/Descision Logic ==
  Disparity : Inport
  Jump : Inport  Port=2
  Frozen : Inport  Port=3
  Partially Frozen : Inport  Port=4
  Enable : Inport  Port=5
  Change Detect : Subsystem
  Latch : Subsystem
  Latch1 : Subsystem
  Logical Operator : Logic  Operator=NOT  AllPortsSameDT=off  OutDataTypeStr=float('double')
  Logical Operator1 : Logic  Inputs=3  AllPortsSameDT=off  OutDataTypeStr=float('double')
  Logical Operator2 : Logic  Inputs=3  AllPortsSameDT=off  OutDataTypeStr=float('double')
  Logical Operator3 : Logic  Operator=OR  AllPortsSameDT=off  OutDataTypeStr=float('double')
  Logical Operator4 : Logic  Operator=OR  AllPortsSameDT=off  OutDataTypeStr=float('double')
  Logical Operator5 : Logic  Operator=NOT  AllPortsSameDT=off  OutDataTypeStr=float('double')
  Logical Operator6 : Logic  AllPortsSameDT=off  OutDataTypeStr=float('double')
  Logical Operator7 : Logic  Operator=NOT  AllPortsSameDT=off  OutDataTypeStr=float('double')
  Logical Operator8 : Logic  Inputs=3  AllPortsSameDT=off  OutDataTypeStr=float('double')
  Memory3 : Memory  InheritSampleTime=on
  Best Bet : Outport
  Fault : Outport  Port=2
  wires:
  Latch1/1(Triggered) -> Logical Operator4/1, Logical Operator5/1
  Frozen/1 -> Logical Operator1/3
  Partially Frozen/1 -> Logical Operator2/3
  Logical Operator3/1 -> Latch1/1(Trigger)
  Logical Operator1/1 -> Logical Operator3/1
  Logical Operator2/1 -> Logical Operator3/2
  Latch/1(Triggered) -> Logical Operator/1, Logical Operator4/2
  Logical Operator/1 -> Logical Operator1/2, Logical Operator2/2
  Logical Operator4/1 -> Fault/1
  Logical Operator5/1 -> Best Bet/1
  Enable/1 -> Memory3/1, Change Detect/2(2), Logical Operator6/1, Logical Operator8/1
  Memory3/1 -> Change Detect/1(1)
  Jump/1 -> Logical Operator6/2
  Change Detect/1(Out) -> Logical Operator7/1
  Logical Operator8/1 -> Logical Operator1/1, Logical Operator2/1
  Logical Operator7/1 -> Logical Operator8/2
  Disparity/1 -> Logical Operator8/3
  Logical Operator6/1 -> Latch/1(Trigger)

== system p1_standalone/Hardware I//O/Input/Handwheel Scaling & Initialization/Handwheel Sensor Fault Detection/Enable Timer ==
  Clock : Clock
  Constant : Constant
  Relational Operator : RelationalOperator  Operator=>  OutDataTypeStr=float('double')
  Enable : Outport
  wires:
  Clock/1 -> Relational Operator/1
  Constant/1 -> Relational Operator/2
  Relational Operator/1 -> Enable/1

== system p1_standalone/Hardware I//O/Input/Handwheel Scaling & Initialization/Handwheel Sensor Fault Detection/Fault Detection1 ==
  Relative : Inport
  Absolute : Inport  Port=2
  Counter : Subsystem
  Counter1 : Subsystem
  Enabled Subsystem : Subsystem  TreatAsAtomicUnit=on
  Enabled Subsystem1 : Subsystem  TreatAsAtomicUnit=on
  Memory : Memory  InheritSampleTime=on
  Memory1 : Memory  InheritSampleTime=on
  Memory2 : Memory  InheritSampleTime=on
  Nearly the Same : Subsystem
  Nearly the Same1 : Subsystem
  Nearly the Same2 : Subsystem
  Nearly the Same3 : Subsystem
  Disparity : Outport
  Jump : Outport  Port=2
  Frozen : Outport  Port=3
  Partially Frozen : Outport  Port=4
  wires:
  Relative/1 -> Nearly the Same3/1(1), Nearly the Same2/1(1), Nearly the Same/2(2), Memory/1
  Absolute/1 -> Nearly the Same3/2(2), Memory2/1, Nearly the Same1/2(2)
  Nearly the Same3/1(Out) -> Disparity/1
  Memory/1 -> Enabled Subsystem/1(In1), Nearly the Same/1(1)
  Enabled Subsystem/1(Out1) -> Memory1/1
  Enabled Subsystem1/1(Out1) -> Nearly the Same2/2(2)
  Memory1/1 -> Enabled Subsystem1/1(In1)
  Counter/1(Time) -> Frozen/1
  Nearly the Same/1(Out) -> Counter/1(In), Enabled Subsystem1/Enable, Enabled Subsystem/Enable
  Nearly the Same2/1(Out) -> Counter1/1(In)
  Counter1/1(Time) -> Partially Frozen/1
  Memory2/1 -> Nearly the Same1/1(1)
  Nearly the Same1/1(Out) -> Jump/1

== system p1_standalone/Hardware I//O/Input/Handwheel Scaling & Initialization/Handwheel Sensor Fault Detection/Switch Over ==
  Relative : Inport
  Chooser : Inport  Port=2
  Absolute : Inport  Port=3
  Logical Operator5 : Logic  Operator=NOT  AllPortsSameDT=off  OutDataTypeStr=float('double')
  Switch : Switch  Threshold=.5
  Switch1 : Switch  Threshold=.5
  Primary : Outport
  Secondary : Outport  Port=2
  wires:
  Switch/1 -> Secondary/1
  Logical Operator5/1 -> Switch1/2
  Relative/1 -> Switch/1, Switch1/1
  Absolute/1 -> Switch/3, Switch1/3
  Switch1/1 -> Primary/1
  Chooser/1 -> Logical Operator5/1, Switch/2

== system p1_standalone/Hardware I//O/Input/OEM4 wgsxyz2enu and status conversion/position preprocessing/Position Converter ==
  xyz : Inport
  reference : Inport  Port=2
  Demux : Demux  Outputs=3
  Mux : Mux  Inputs=2
  S-Function2 : S-Function  FunctionName=wgsxyz2enuP  EnableBusSupport=off
  East(x) : Outport
  North(Y) : Outport  Port=2
  Up : Outport  Port=3
  wires:
  xyz/1 -> Mux/1
  reference/1 -> Mux/2
  Mux/1 -> S-Function2/1
  Demux/3 -> Up/1
  Demux/2 -> North(Y)/1
  Demux/1 -> East(x)/1
  S-Function2/1 -> Demux/1

== system p1_standalone/Hardware I//O/Input/OEM4 wgsxyz2enu and status conversion/velocity preprocessing/Velocity Converter ==
  xyz : Inport
  reference : Inport  Port=2
  Demux : Demux  Outputs=3
  Mux : Mux  Inputs=2
  S-Function2 : S-Function  FunctionName=wgsxyz2enuV  EnableBusSupport=off
  East(x) : Outport
  North(Y) : Outport  Port=2
  Up : Outport  Port=3
  wires:
  xyz/1 -> Mux/1
  reference/1 -> Mux/2
  Mux/1 -> S-Function2/1
  Demux/3 -> Up/1
  Demux/2 -> North(Y)/1
  Demux/1 -> East(x)/1
  S-Function2/1 -> Demux/1

== system p1_standalone/Sensor Data and Estimation/Vehicle State Estimator/state estimation/Super Filter/Accelerometer Pre-Processing ==
  Long Acc (ax) : Inport
  Lat Acc (ay) : Inport  Port=2
  Memory : Memory
  Sum2 : Sum  Inputs=|++  SaturateOnIntegerOverflow=on  InputSameDT=on  OutDataTypeStr=Inherit: Same as first input
  Sum3 : Sum  Inputs=|++  SaturateOnIntegerOverflow=on  InputSameDT=on  OutDataTypeStr=Inherit: Same as first input
  Sum4 : Sum  Inputs=|+-  SaturateOnIntegerOverflow=on  InputSameDT=on  OutDataTypeStr=Inherit: Same as first input
  Sum5 : Sum  Inputs=|+-  SaturateOnIntegerOverflow=on  InputSameDT=on  OutDataTypeStr=Inherit: Same as first input
  ax Bias : Constant  Value=gpsins.long_acc_bias
  ax sf : Gain  Gain=gpsins.long_acc_sf  SaturateOnIntegerOverflow=on  OutDataTypeStr=Inherit: Same as input  ParamDataTypeStr=Inherit: Same as input
  ay Bias : Constant  Value=gpsins.lat_acc_bias
  ay sf : Gain  Gain=gpsins.lat_acc_sf  SaturateOnIntegerOverflow=on  OutDataTypeStr=Inherit: Same as input  ParamDataTypeStr=Inherit: Same as input
  cross coupling from ax : Gain  Gain=gpsins.long_to_lat  SaturateOnIntegerOverflow=on  OutDataTypeStr=Inherit: Same as input  ParamDataTypeStr=Inherit: Same as input
  cross coupling from ay : Gain  Gain=gpsins.lat_to_long  SaturateOnIntegerOverflow=on  OutDataTypeStr=Inherit: Same as input  ParamDataTypeStr=Inherit: Same as input
  ax : Outport
  ay : Outport  Port=2
  wires:
  Memory/1 -> cross coupling from ax/1
  Sum4/1 -> Memory/1, ax/1
  Sum5/1 -> cross coupling from ay/1, ay/1
  ay sf/1 -> Sum5/1
  cross coupling from ax/1 -> Sum5/2
  ax sf/1 -> Sum4/1
  cross coupling from ay/1 -> Sum4/2
  Long Acc (ax)/1 -> Sum3/1
  Sum3/1 -> ax sf/1
  ax Bias/1 -> Sum3/2
  Sum2/1 -> ay sf/1
  Lat Acc (ay)/1 -> Sum2/1
  ay Bias/1 -> Sum2/2
